simulink model "ketszereplos"  (Simulink 7.8)
settings: Solver=ode45  StartTime=0.0  StopTime=10.0  RelTol=1e-3
settings Model: Creator=valaki  LastModifiedBy=valaki

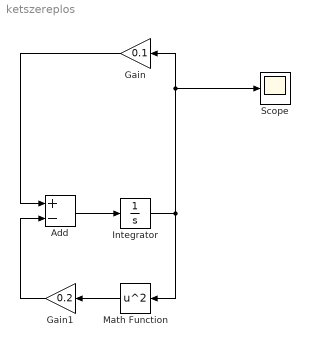
== system ketszereplos ==
  Add : Sum  Inputs=+-
  Gain : Gain  Gain=0.1
  Gain1 : Gain  Gain=0.2
  Integrator : Integrator  InitialCondition=0.2
  Math Function : Math  Operator=square  SaturateOnIntegerOverflow=on
  Scope : Scope
  wires:
  Integrator/1 -> Gain/1, Scope/1, Math Function/1
  Math Function/1 -> Gain1/1
  Gain/1 -> Add/1
  Gain1/1 -> Add/2
  Add/1 -> Integrator/1
